simulink model "partThreeDifferentialDrive"  (R2021b)
settings: Solver=VariableStepAuto  StartTime=0.0  StopTime=50  RelTol=1e-3
settings Model: Creator=ericp  LastModifiedBy=ericp

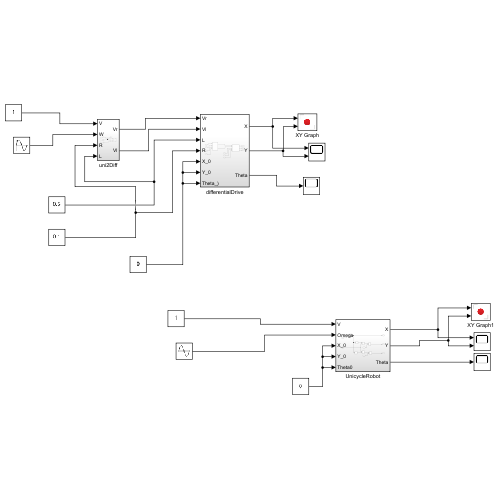
[thumbnail: Simulink's stored preview of the top-level diagram]
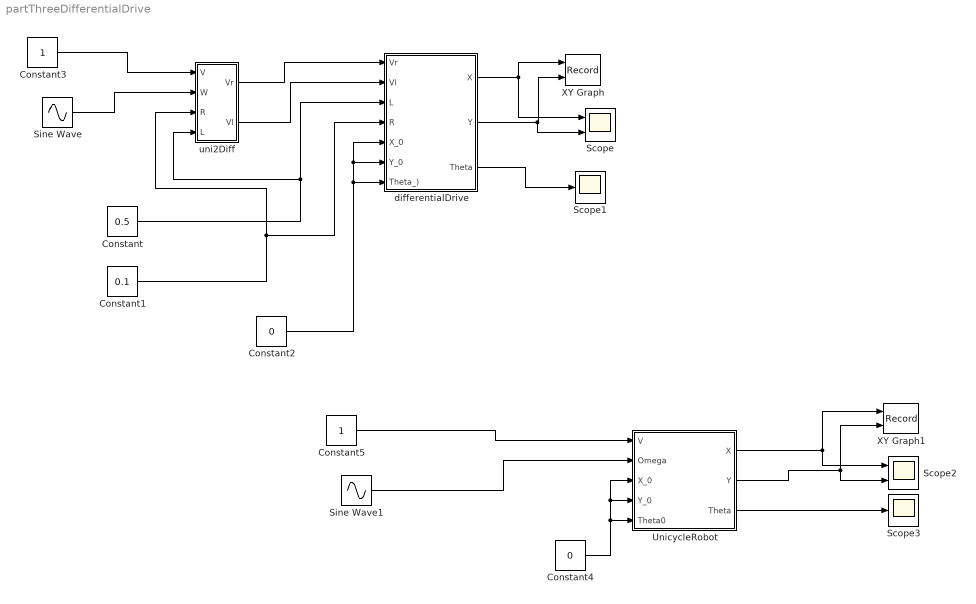
== system partThreeDifferentialDrive ==
  Constant : Constant  Value=0.5
  Constant1 : Constant  Value=0.1
  Constant2 : Constant  Value=0
  Constant3 : Constant
  Constant4 : Constant  Value=0
  Constant5 : Constant
  Scope : Scope  NumInputPorts=2
  Scope1 : Scope
  Scope2 : Scope  NumInputPorts=2
  Scope3 : Scope
  Sine Wave : Sin  Frequency=100  SampleTime=0
  Sine Wave1 : Sin  Frequency=100  SampleTime=0
  UnicycleRobot : Subsystem
  XY Graph : Record  FileSettingsInternal="{\"entries\":[{\"content\":{\"excelSettings\":{\"content\":{},\"type\":\"Streamout.ExcelSettings\"}},\"type\":\"Streamout.FileSettingStorage\",\"uuid\":\"c3335ff7-5187-4557-909c-4a25491fdaa3\"}],\"packageUris\":[\"http://schema.mathworks.com/mf0/streamout_blocks/R2020a\"],\"version\":\"1.0\"}"  Layout=[1 1]  SignalsInternal="{\"entries\":[{\"content\":{\"signals\":[{\"content\":{\"blockPath\":[\"partThreeDifferentialDrive/XY Graph\"],\"channel\":[],\"dimensions\":[1],\"domain\":\"partThreeDifferentialDrive/XY Graph\",\"lineColor\":\"#ff6929\",\"plots\":[],\"port\":1,\"sid\":[\"\"],\"signalID\":45,\"signalName\":\"differentialDrive:1\"},\"type\":\"RecordBlkView.Signal\",\"uuid\":\"d0da75a7-5d7c-4b87-8c11-277256da90d9\"},{\"content\":{\"blockPath\":[\"partThreeDifferentialDrive/XY Graph\"],\"channel\":[],\"dimensions\":[1],\"domain\":\"partThreeDifferentialDrive/XY Graph\",\"lineColor\":\"#b746ff\",\"plots\":[1],\"port\":2,\"sid\":[\"\"],\"signalID\":49,\"signalName\":\"differentialDrive:2\"},\"type\":\"RecordBlkView.Signal\",\"uuid\":\"7e01b0ac-52c4-48b3-b27d-7a93332c5813\"}]},\"type\":\"RecordBlkView.InputSignals\",\"uuid\":\"04b5fb78-b9c1-406f-a8ac-25f42f337439\"}],\"packageUris\":[\"http://schema.mathworks.com/mf0/streamout_blocks/R2020a\"],\"version\":\"1.0\"}"  VisualizationBindings="{\"xyplotplugin\":{\"info\":[{\"series\":[],\"subplotID\":1}]}}"  CompatibilityTag=XY
  XY Graph1 : Record  FileSettingsInternal="{\"entries\":[{\"content\":{\"excelSettings\":{\"content\":{},\"type\":\"Streamout.ExcelSettings\"}},\"type\":\"Streamout.FileSettingStorage\",\"uuid\":\"ca527cc9-686f-4f9e-b3db-7a451a1c4e36\"}],\"packageUris\":[\"http://schema.mathworks.com/mf0/streamout_blocks/R2020a\"],\"version\":\"1.0\"}"  Layout=[1 1]  SignalsInternal="{\"entries\":[{\"content\":{\"signals\":[{\"content\":{\"blockPath\":[\"partThreeDifferentialDrive/XY Graph1\"],\"channel\":[],\"dimensions\":[1],\"domain\":\"partThreeDifferentialDrive/XY Graph1\",\"lineColor\":\"#a2142f\",\"plots\":[1],\"port\":1,\"sid\":[\"\"],\"signalID\":53,\"signalName\":\"UnicycleRobot:1\"},\"type\":\"RecordBlkView.Signal\",\"uuid\":\"929b2522-787c-47b8-8d58-de7029b9b016\"},{\"content\":{\"blockPath\":[\"partThreeDifferentialDrive/XY Graph1\"],\"channel\":[],\"dimensions\":[1],\"domain\":\"partThreeDifferentialDrive/XY Graph1\",\"lineColor\":\"#139fff\",\"plots\":[1],\"port\":2,\"sid\":[\"\"],\"signalID\":57,\"signalName\":\"UnicycleRobot:2\"},\"type\":\"RecordBlkView.Signal\",\"uuid\":\"cb2d85a0-4790-4687-90f3-ef2b0f1a3a33\"}]},\"type\":\"RecordBlkView.InputSignals\",\"uuid\":\"ef842469-8e91-4726-9b0f-1f7d87fcc339\"}],\"packageUris\":[\"http://schema.mathworks.com/mf0/streamout_blocks/R2020a\"],\"version\":\"1.0\"}"  VisualizationBindings="{\"xyplotplugin\":{\"info\":[{\"series\":[{\"bindingParametersList\":[{\"parameter\":\"X-Axis\",\"signalID\":57,\"signalName\":\"UnicycleRobot:2\"},{\"parameter\":\"Y-Axis\",\"signalID\":53,\"signalName\":\"UnicycleRobot:1\"}],\"seriesID\":27540}],\"subplotID\":1}]}}"  CompatibilityTag=XY
  differentialDrive : Subsystem
  uni2Diff : Subsystem
  wires:
  Constant1/1 -> uni2Diff/3(R), differentialDrive/4(R)
  uni2Diff/1(Vr) -> differentialDrive/1(Vr)
  uni2Diff/2(Vl) -> differentialDrive/2(Vl)
  Constant/1 -> uni2Diff/4(L), differentialDrive/3(L)
  Constant2/1 -> differentialDrive/6(Y_0), differentialDrive/5(X_0), differentialDrive/7(Theta_))
  Constant3/1 -> uni2Diff/1(V)
  Sine Wave/1 -> uni2Diff/2(W)
  differentialDrive/1(X) -> XY Graph/1, Scope/1
  differentialDrive/2(Y) -> Scope/2, XY Graph/2
  differentialDrive/3(Theta) -> Scope1/1
  Sine Wave1/1 -> UnicycleRobot/2(Omega)
  Constant4/1 -> UnicycleRobot/5(Theta0), UnicycleRobot/4(Y_0), UnicycleRobot/3(X_0)
  UnicycleRobot/2(Y) -> XY Graph1/2, Scope2/2
  Constant5/1 -> UnicycleRobot/1(V)
  UnicycleRobot/1(X) -> XY Graph1/1, Scope2/1
  UnicycleRobot/3(Theta) -> Scope3/1

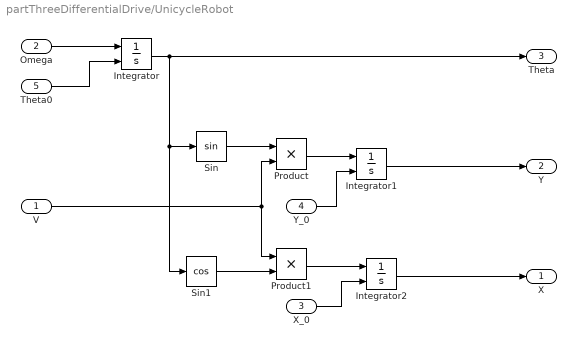
== system partThreeDifferentialDrive/UnicycleRobot ==
  V : Inport
  Omega : Inport  Port=2
  X_0 : Inport  Port=3
  Y_0 : Inport  Port=4
  Theta0 : Inport  Port=5
  Integrator : Integrator  InitialConditionSource=external
  Integrator1 : Integrator  InitialConditionSource=external
  Integrator2 : Integrator  InitialConditionSource=external
  Product : Product
  Product1 : Product
  Sin : Trigonometry
  Sin1 : Trigonometry  Operator=cos
  X : Outport
  Y : Outport  Port=2
  Theta : Outport  Port=3
  wires:
  Sin1/1 -> Product1/2
  V/1 -> Product1/1, Product/2
  Integrator/1 -> Theta/1, Sin1/1, Sin/1
  Integrator2/1 -> X/1
  Sin/1 -> Product/1
  Theta0/1 -> Integrator/2
  Y_0/1 -> Integrator1/2
  Omega/1 -> Integrator/1
  X_0/1 -> Integrator2/2
  Integrator1/1 -> Y/1
  Product1/1 -> Integrator2/1
  Product/1 -> Integrator1/1

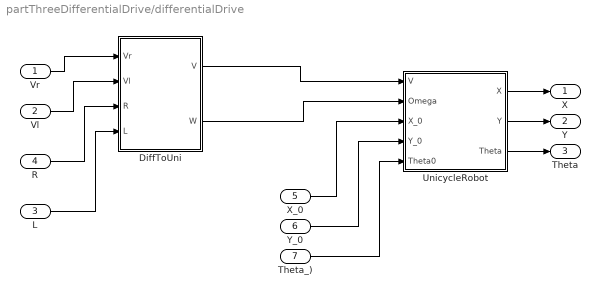
== system partThreeDifferentialDrive/differentialDrive ==
  Vr : Inport
  Vl : Inport  Port=2
  L : Inport  Port=3
  R : Inport  Port=4
  X_0 : Inport  Port=5
  Y_0 : Inport  Port=6
  Theta_) : Inport  Port=7
  DiffToUni : Subsystem
  UnicycleRobot : Subsystem
  X : Outport
  Y : Outport  Port=2
  Theta : Outport  Port=3
  wires:
  Y_0/1 -> UnicycleRobot/4(Y_0)
  UnicycleRobot/3(Theta) -> Theta/1
  UnicycleRobot/1(X) -> X/1
  UnicycleRobot/2(Y) -> Y/1
  DiffToUni/1(V) -> UnicycleRobot/1(V)
  Theta_)/1 -> UnicycleRobot/5(Theta0)
  Vr/1 -> DiffToUni/1(Vr)
  DiffToUni/2(W) -> UnicycleRobot/2(Omega)
  R/1 -> DiffToUni/3(R)
  Vl/1 -> DiffToUni/2(Vl)
  L/1 -> DiffToUni/4(L)
  X_0/1 -> UnicycleRobot/3(X_0)

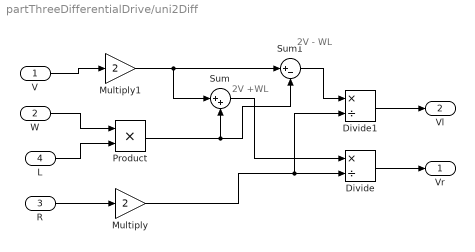
== system partThreeDifferentialDrive/uni2Diff ==
  note: 2V +WL
  note: 2V - WL
  V : Inport
  W : Inport  Port=2
  R : Inport  Port=3
  L : Inport  Port=4
  Divide : Product  Inputs=*/
  Divide1 : Product  Inputs=*/
  Multiply : Gain  Gain=2
  Multiply1 : Gain  Gain=2
  Product : Product
  Sum : Sum  Inputs=|++
  Sum1 : Sum  Inputs=|+-
  Vr : Outport
  Vl : Outport  Port=2
  wires:
  V/1 -> Multiply1/1
  Divide/1 -> Vr/1
  Sum1/1 -> Divide1/1
  Multiply/1 -> Divide1/2, Divide/2
  Divide1/1 -> Vl/1
  L/1 -> Product/2
  R/1 -> Multiply/1
  Multiply1/1 -> Sum1/1, Sum/1
  Sum/1 -> Divide/1
  Product/1 -> Sum1/2, Sum/2
  W/1 -> Product/1

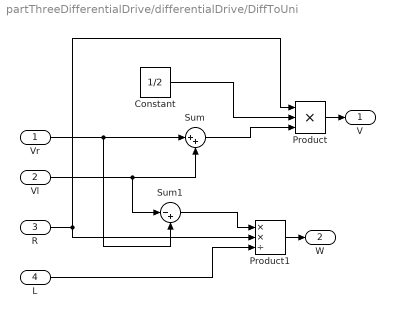
== system partThreeDifferentialDrive/differentialDrive/DiffToUni ==
  Vr : Inport
  Vl : Inport  Port=2
  R : Inport  Port=3
  L : Inport  Port=4
  Constant : Constant  Value=1/2
  Product : Product  Inputs=3
  Product1 : Product  Inputs=**/  InputSameDT=on
  Sum : Sum  Inputs=|++
  Sum1 : Sum  Inputs=|-+
  V : Outport
  W : Outport  Port=2
  wires:
  Vl/1 -> Sum1/1, Sum/2
  L/1 -> Product1/3
  Sum/1 -> Product/3
  Vr/1 -> Sum1/2, Sum/1
  R/1 -> Product1/2, Product/1
  Constant/1 -> Product/2
  Sum1/1 -> Product1/1
  Product/1 -> V/1
  Product1/1 -> W/1

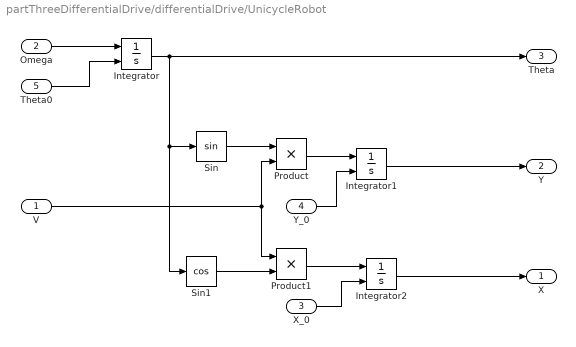
== system partThreeDifferentialDrive/differentialDrive/UnicycleRobot ==
  V : Inport
  Omega : Inport  Port=2
  X_0 : Inport  Port=3
  Y_0 : Inport  Port=4
  Theta0 : Inport  Port=5
  Integrator : Integrator  InitialConditionSource=external
  Integrator1 : Integrator  InitialConditionSource=external
  Integrator2 : Integrator  InitialConditionSource=external
  Product : Product
  Product1 : Product
  Sin : Trigonometry
  Sin1 : Trigonometry  Operator=cos
  X : Outport
  Y : Outport  Port=2
  Theta : Outport  Port=3
  wires:
  Sin1/1 -> Product1/2
  V/1 -> Product1/1, Product/2
  Integrator/1 -> Theta/1, Sin1/1, Sin/1
  Integrator2/1 -> X/1
  Sin/1 -> Product/1
  Theta0/1 -> Integrator/2
  Y_0/1 -> Integrator1/2
  Omega/1 -> Integrator/1
  X_0/1 -> Integrator2/2
  Integrator1/1 -> Y/1
  Product1/1 -> Integrator2/1
  Product/1 -> Integrator1/1
